simulink model "Robot_control"  (R2021b)
settings: Solver=FixedStepAuto  StartTime=0.0  StopTime=6.5  FixedStep=0.001  RelTol=1e-5  AbsTol=1e-4
values from neighbouring files (symbols this model uses):
  CtlSat1 = CtlSat(1)    [constants.m]
  CtlSat2 = CtlSat(2)    [constants.m]
  CtlSat3 = CtlSat(3)    [constants.m]
  CtlSat4 = CtlSat(4)    [constants.m]
  CtlSat5 = CtlSat(5)    [constants.m]
  CtlSat6 = CtlSat(6)    [constants.m]
  goal_point = [10;-75;10;10;10;10]*pi/180    [constants.m]
  KP = [8,zeros(1,5);0,7,zeros(1,4);0,0,7,zeros(1,3);zeros(1,3),5,0,0;zeros(1,4),4,0;zeros(1,5),2]    [constants.m]
  KV = [4,zeros(1,5);0,8,zeros(1,4);0,0,7,zeros(1,3);zeros(1,3),5,0,0;zeros(1,4),4,0;zeros(1,5),2]    [constants.m]
  speed_goal = [10;10;10;4;2;9]*pi/180    [constants.m]
settings Model: Creator=zhikai  LastModifiedBy=zhikai

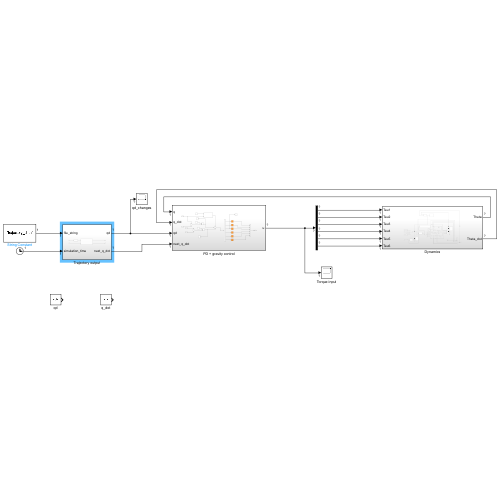
[thumbnail: Simulink's stored preview of the top-level diagram]
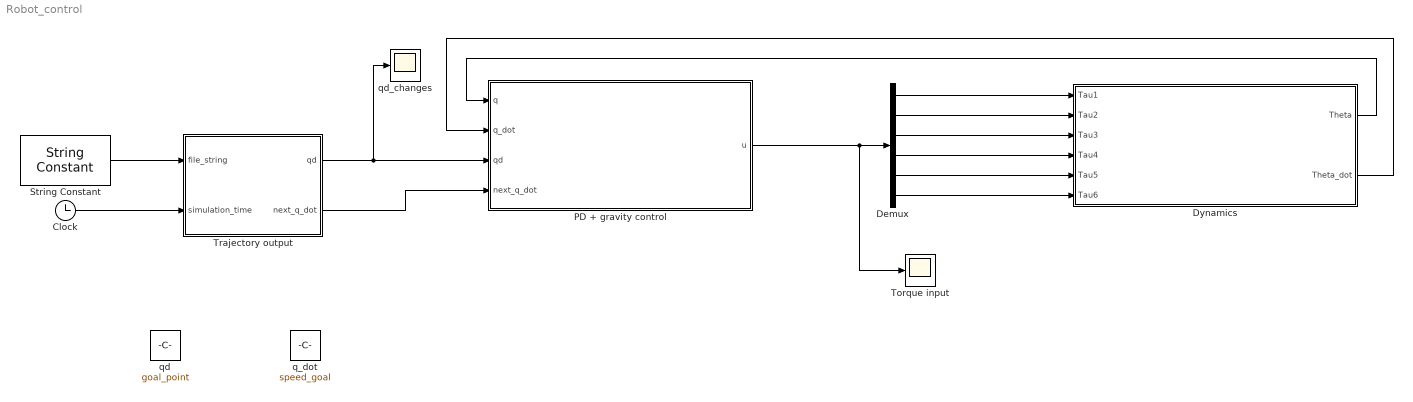
== system Robot_control ==
  Clock : Clock
  Demux : Demux  Outputs=6
  Dynamics : Subsystem
  PD + gravity control : Subsystem
  String Constant : StringConstant  String="\"trajectory_data\""
  Torque input : Scope
  Trajectory output : Subsystem
  q_dot : Constant  Value=speed_goal
  qd : Constant  Value=goal_point
  qd_changes : Scope
  wires:
  Dynamics/1(Theta) -> PD + gravity control/1(q)
  Dynamics/2(Theta_dot) -> PD + gravity control/2(q_dot)
  PD + gravity control/1(u) -> Torque input/1, Demux/1
  Demux/3 -> Dynamics/3(Tau3)
  Demux/6 -> Dynamics/6(Tau6)
  Demux/4 -> Dynamics/4(Tau4)
  Demux/2 -> Dynamics/2(Tau2)
  Demux/1 -> Dynamics/1(Tau1)
  Demux/5 -> Dynamics/5(Tau5)
  Trajectory output/1(qd) -> qd_changes/1, PD + gravity control/3(qd)
  Trajectory output/2(next_q_dot) -> PD + gravity control/4(next_q_dot)
  String Constant/1 -> Trajectory output/1(file_string)
  Clock/1 -> Trajectory output/2(simulation_time)

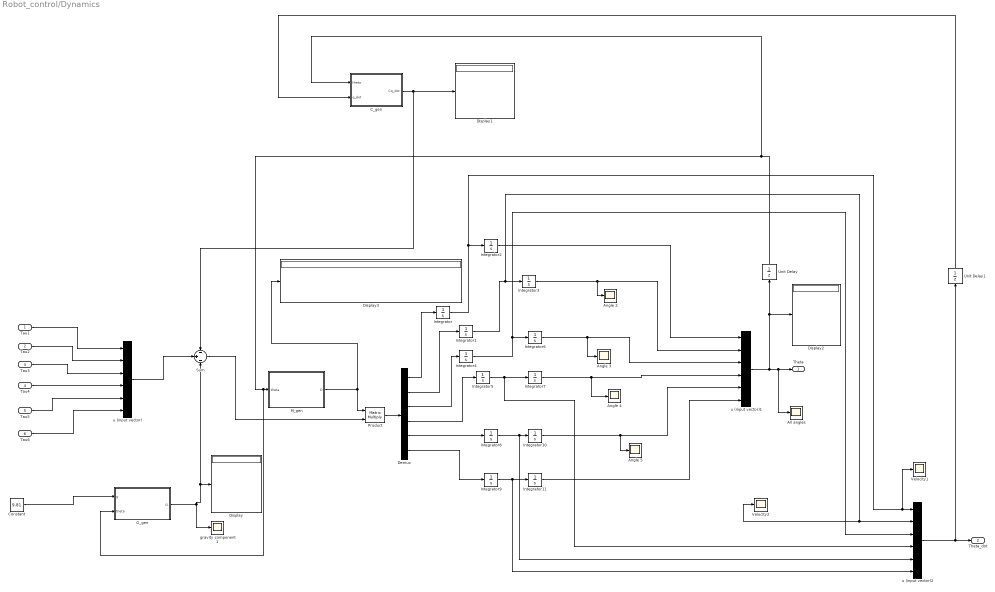
== system Robot_control/Dynamics ==
  Tau1 : Inport
  Tau2 : Inport  Port=2
  Tau3 : Inport  Port=3
  Tau4 : Inport  Port=4
  Tau5 : Inport  Port=5
  Tau6 : Inport  Port=6
  All angles : Scope
  Angle {2..5} (4 alike) : Scope
  C_gen : MATLAB Function  TreatAsAtomicUnit=on
  Constant : Constant  Value=9.81
  Demux : Demux  Outputs=6
  Display{,1..3} (4 alike) : Display
      Display settings: Decimation=6
      Display1 settings: Decimation=6
      Display2 settings: Decimation=6
      Display3 settings: Decimation=36
  G_gen : MATLAB Function  TreatAsAtomicUnit=on
  Integrator{,1..11} (12 alike) : Integrator
  M_gen : MATLAB Function  TreatAsAtomicUnit=on
  Product : Product  Multiplication=Matrix(*)
  Sum : Sum  Inputs=-|+|-
  Unit Delay : UnitDelay  InitialCondition=[-pi/2;0;0;0;0;0]  SampleTime=-1  HasFrameUpgradeWarning=on
  Unit Delay1 : UnitDelay  InitialCondition=[0;0;0;0;0;0]  SampleTime=-1  HasFrameUpgradeWarning=on
  Velocity1 : Scope
  Velocity2 : Scope
  gravity component 1 : Scope
  u (input vector) : Concatenate  NumInputs=6
  u (input vector)1 : Concatenate  NumInputs=6
  u (input vector)2 : Concatenate  NumInputs=6
  Theta : Outport  VectorParamsAs1DForOutWhenUnconnected=off
  Theta_dot : Outport  Port=2  VectorParamsAs1DForOutWhenUnconnected=off
  wires:
  Demux/4 -> Integrator5/1
  M_gen/1(D) -> Product/1, Display3/1
  Integrator6/1 -> Angle 3/1, u (input vector)1/3
  Unit Delay/1 -> C_gen/1(theta), G_gen/2(theta), M_gen/1(theta)
  Tau5/1 -> u (input vector)/5
  Integrator3/1 -> Angle 2/1, u (input vector)1/2
  u (input vector)2/1 -> Unit Delay1/1, Theta_dot/1
  C_gen/1(Cq_dot) -> Display1/1, Sum/1
  u (input vector)/1 -> Sum/2
  u (input vector)1/1 -> Unit Delay/1, Display2/1, All angles/1, Theta/1
  Integrator8/1 -> u (input vector)2/5, Integrator10/1
  Integrator4/1 -> Integrator6/1, u (input vector)2/3
  Demux/5 -> Integrator8/1
  Integrator2/1 -> u (input vector)1/1
  Integrator7/1 -> Angle 4/1, u (input vector)1/4
  Demux/3 -> Integrator4/1
  Integrator11/1 -> u (input vector)1/6
  Integrator/1 -> Integrator2/1, Velocity1/1, u (input vector)2/1
  Demux/6 -> Integrator9/1
  Constant/1 -> G_gen/1(g)
  Integrator9/1 -> u (input vector)2/6, Integrator11/1
  Tau1/1 -> u (input vector)/1
  Tau6/1 -> u (input vector)/6
  Integrator1/1 -> Integrator3/1, u (input vector)2/2, Velocity2/1
  G_gen/1(G) -> Sum/3, Display/1, gravity component 1/1
  Integrator5/1 -> u (input vector)2/4, Integrator7/1
  Demux/2 -> Integrator1/1
  Sum/1 -> Product/2
  Tau3/1 -> u (input vector)/3
  Tau4/1 -> u (input vector)/4
  Demux/1 -> Integrator/1
  Tau2/1 -> u (input vector)/2
  Integrator10/1 -> Angle 5/1, u (input vector)1/5
  Product/1 -> Demux/1
  Unit Delay1/1 -> C_gen/2(q_dot)

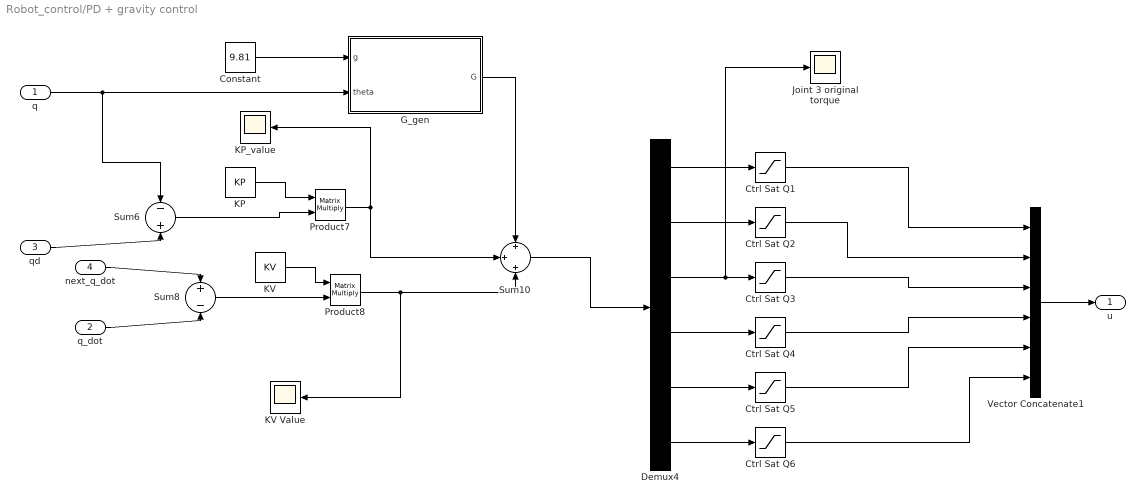
== system Robot_control/PD + gravity control ==
  q : Inport
  q_dot : Inport  Port=2
  qd : Inport  Port=3
  next_q_dot : Inport  Port=4
  Constant : Constant  Value=9.81
  Ctrl Sat Q1 : Saturate  UpperLimit=CtlSat1  LowerLimit=-CtlSat1
  Ctrl Sat Q2 : Saturate  UpperLimit=CtlSat2  LowerLimit=-CtlSat2
  Ctrl Sat Q3 : Saturate  UpperLimit=CtlSat3  LowerLimit=-CtlSat3
  Ctrl Sat Q4 : Saturate  UpperLimit=CtlSat4  LowerLimit=-CtlSat4
  Ctrl Sat Q5 : Saturate  UpperLimit=CtlSat5  LowerLimit=-CtlSat5
  Ctrl Sat Q6 : Saturate  UpperLimit=CtlSat6  LowerLimit=-CtlSat6
  Demux4 : Demux  Outputs=6
  G_gen : MATLAB Function  TreatAsAtomicUnit=on
  Joint 3 original torque : Scope
  KP : Constant  Value=KP
  KP_value : Scope
  KV : Constant  Value=KV
  "KV Value " : Scope
  Product7 : Product  Multiplication=Matrix(*)
  Product8 : Product  Multiplication=Matrix(*)
  Sum10 : Sum  Inputs=+|+|+
  Sum6 : Sum  Inputs=-|+
  Sum8 : Sum  Inputs=+|-
  Vector Concatenate1 : Concatenate  NumInputs=6
  u : Outport  VectorParamsAs1DForOutWhenUnconnected=off
  wires:
  Sum8/1 -> Product8/2
  KP/1 -> Product7/1
  Product8/1 -> "KV Value "/1, Sum10/3
  qd/1 -> Sum6/2
  Product7/1 -> KP_value/1, Sum10/2
  q_dot/1 -> Sum8/2
  Sum6/1 -> Product7/2
  q/1 -> G_gen/2(theta), Sum6/1
  next_q_dot/1 -> Sum8/1
  KV/1 -> Product8/1
  Constant/1 -> G_gen/1(g)
  G_gen/1(G) -> Sum10/1
  Sum10/1 -> Demux4/1
  Demux4/1 -> Ctrl Sat Q1/1
  Demux4/2 -> Ctrl Sat Q2/1
  Demux4/3 -> Joint 3 original torque/1, Ctrl Sat Q3/1
  Demux4/4 -> Ctrl Sat Q4/1
  Demux4/5 -> Ctrl Sat Q5/1
  Demux4/6 -> Ctrl Sat Q6/1
  Vector Concatenate1/1 -> u/1
  Ctrl Sat Q1/1 -> Vector Concatenate1/1
  Ctrl Sat Q2/1 -> Vector Concatenate1/2
  Ctrl Sat Q3/1 -> Vector Concatenate1/3
  Ctrl Sat Q4/1 -> Vector Concatenate1/4
  Ctrl Sat Q5/1 -> Vector Concatenate1/5
  Ctrl Sat Q6/1 -> Vector Concatenate1/6

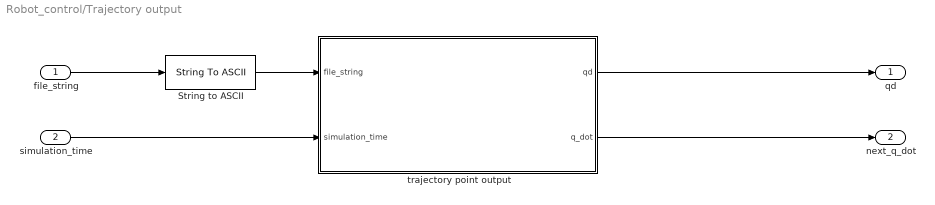
== system Robot_control/Trajectory output ==
  file_string : Inport
  simulation_time : Inport  Port=2
  String to ASCII : StringToASCII
  trajectory point output : MATLAB Function  TreatAsAtomicUnit=on
  qd : Outport  VectorParamsAs1DForOutWhenUnconnected=off
  next_q_dot : Outport  Port=2  VectorParamsAs1DForOutWhenUnconnected=off
  wires:
  trajectory point output/1(qd) -> qd/1
  trajectory point output/2(q_dot) -> next_q_dot/1
  simulation_time/1 -> trajectory point output/2(simulation_time)
  file_string/1 -> String to ASCII/1
  String to ASCII/1 -> trajectory point output/1(file_string)

== matlab function Robot_control/Dynamics/C_gen ==
  data: theta input; Cq_dot output; q_dot input
function Cq_dot = Get_Cq_dot(theta,   q_dot)
    Cq_dot = zeros(6,1);
    eml.extrinsic('C_gen');
    C_temp = C_gen(theta, q_dot);
    Cq_dot = C_temp*q_dot;
end

== matlab function Robot_control/Dynamics/M_gen ==
  data: theta input; D output
function D = Get_M(theta)
   D = zeros(6,6);
   coder.extrinsic('D_gen');
   D_temp = D_gen(theta);
   D = inv(D_temp);
   %D = D + J_rotor;
end

== matlab function Robot_control/PD + gravity control/G_gen ==
  data: g input; G output; theta input
function G = Get_G( g, theta)
    G = zeros(6,1);
    eml.extrinsic('G_gen');
    G = G_gen(g,theta);
end

== matlab function Robot_control/Trajectory output/trajectory point output ==
  data: file_string input; qd output size=6,1; q_dot output size=6,1; simulation_time input
function [qd, q_dot] = fcn(file_string, simulation_time)
    %#codegen
    %traj_data = [time, pos (1x6), vel(1x6)]
    trajectory_index = 0;
    file_string = char(file_string)
    data_size = zeros(1,2);
    coder.extrinsic("trajectory_size");
    coder.extrinsic("trajectory_output");
    data_size = trajectory_size(file_string);
    data_all = zeros(data_size(1), data_size(2));
    data_all = trajectory_output(file_string);
    %time = get_param('Robot_control','SimulationTime');
    %disp(simulation_time)
    data_time_size = size(data_all, 1);
    data_time = data_all(1:data_time_size, 1) - data_all(1);
    disp(data_time);
    trajectory_index = find( data_time > simulation_time, 1 );
    qd = reshape(data_all(trajectory_index, 2:7), 6,1);
    q_dot = reshape(data_all(trajectory_index, 8:size(data_all, 2)), 6,1);
    %num_time_stamps = (data_time(length(data_time))-data_time(1))/length(data_time);

end

== matlab function Robot_control/Dynamics/G_gen ==
  data: g input; G output; theta input
function G = Get_G( g, theta)
    G = zeros(6,1);
    eml.extrinsic('G_gen');
    G = G_gen(g,theta);
end
